simulink model "envelope_demodulation"  (R2019b)
settings: Solver=VariableStepAuto  StartTime=0.0  StopTime=0.008  RelTol=1e-3
undefined symbols (not defined in the file): magnitude
libraries: dsparch4 x1
settings Model: Creator=Lenovo  LastModifiedBy=Lenovo

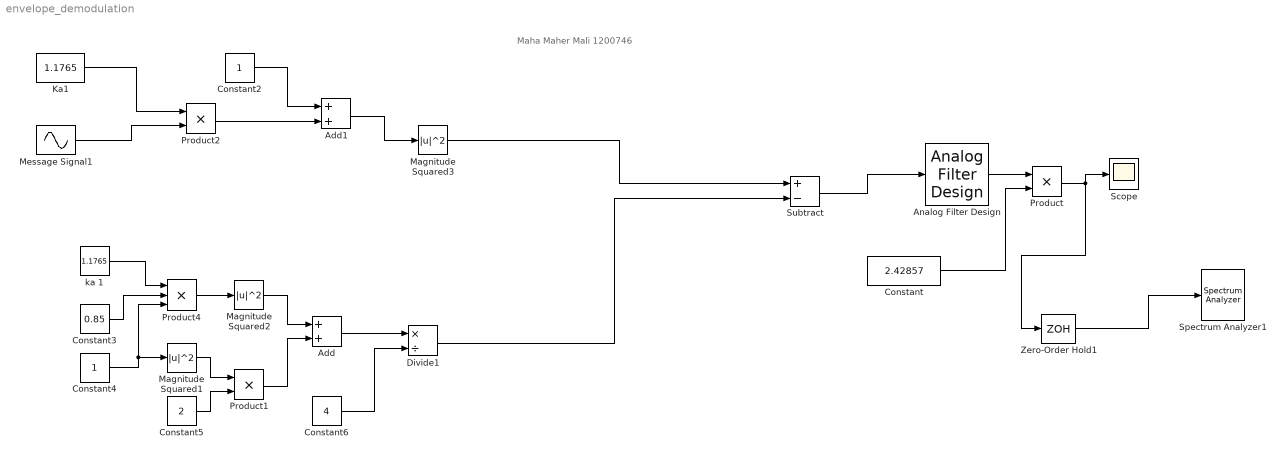
== system envelope_demodulation ==
  note: Maha Maher Mali 1200746
  Add : Sum
  Add1 : Sum
  Analog Filter Design : dsparch4/Analog Filter Design  method=Butterworth  filttype=Lowpass  N=8  Wlo=2*pi*1200  Whi=80  Rp=2  Rs=40
  Constant : Constant  Value=2.42857
  Constant2 : Constant
  Constant3 : Constant  Value=0.85
  Constant4 : Constant
  Constant5 : Constant  Value=2
  Constant6 : Constant  Value=4
  Divide1 : Product  Inputs=*/
  Ka1 : Constant  Value=1.1765
  Magnitude Squared1 : Math  Operator=magnitude^2  SignedPower=off  SaturateOnIntegerOverflow=on
  Magnitude Squared2 : Math  Operator=magnitude^2  SignedPower=off  SaturateOnIntegerOverflow=on
  Magnitude Squared3 : Math  Operator=magnitude^2  SignedPower=off  SaturateOnIntegerOverflow=on
  Message Signal1 : Sin  Amplitude=0.85  Frequency=2*pi*1000  SampleTime=0
  Product : Product
  Product1 : Product
  Product2 : Product
  Product4 : Product  Inputs=3
  Scope : Scope
  Spectrum Analyzer1 : SpectrumAnalyzer
  Subtract : Sum  Inputs=+-
  Zero-Order Hold1 : ZeroOrderHold  SampleTime=1/(10*1e3)
  ka 1 : Constant  Value=1.1765
  wires:
  Subtract/1 -> Analog Filter Design/1
  Product1/1 -> Add/2
  Magnitude Squared1/1 -> Product1/1
  Constant5/1 -> Product1/2
  Magnitude Squared2/1 -> Add/1
  Constant6/1 -> Divide1/2
  Add/1 -> Divide1/1
  Product4/1 -> Magnitude Squared2/1
  Constant4/1 -> Magnitude Squared1/1, Product4/3
  Constant3/1 -> Product4/2
  ka 1/1 -> Product4/1
  Divide1/1 -> Subtract/2
  Zero-Order Hold1/1 -> Spectrum Analyzer1/1
  Product2/1 -> Add1/2
  Message Signal1/1 -> Product2/2
  Ka1/1 -> Product2/1
  Constant2/1 -> Add1/1
  Magnitude Squared3/1 -> Subtract/1
  Add1/1 -> Magnitude Squared3/1
  Analog Filter Design/1 -> Product/1
  Constant/1 -> Product/2
  Product/1 -> Scope/1, Zero-Order Hold1/1
